simulink model "test_crypto_pc"  (R2019b)
settings: Solver=FixedStepAuto  StartTime=0.0  StopTime=20  FixedStep=0.0001  RelTol=1e-3
settings Model: Creator=Oboe  LastModifiedBy=Luca

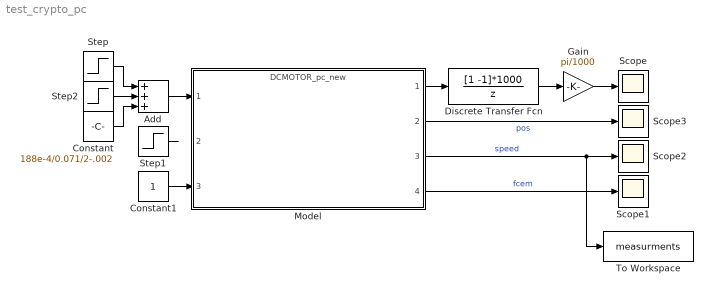
== system test_crypto_pc ==
  Add : Sum  Inputs=+++
  Constant : Constant  Value=188e-4/0.071/2-.002
  Constant1 : Constant
  Discrete Transfer Fcn : DiscreteTransferFcn  Numerator=[1 -1]*1000  Denominator=[1 0]  SampleTime=.001
  Gain : Gain  Gain=pi/1000
  Model : ModelReference  ModelNameDialog=DCMOTOR_pc_new.slxp  ModelReferenceVersion=1.21  CopyOfModelProtected=on
  Scope{,1..3} (4 alike) : Scope
  Step : Step  After=.5  SampleTime=0
  Step1 : Step  Time=10  After=-.5  SampleTime=0
  Step2 : Step  Time=10  After=-0.5  SampleTime=0
  To Workspace : ToWorkspace  VariableName=measurments  SaveFormat=Structure With Time  SampleTime=-1
      settings: Decimation=100
  wires:
  Model/1 -> Discrete Transfer Fcn/1
  Discrete Transfer Fcn/1 -> Gain/1
  Gain/1 -> Scope/1
  Model/4 -> Scope1/1  "fcem"
  Step/1 -> Add/1
  Constant/1 -> Add/3
  Step1/1 -> ?
  Model/2 -> Scope3/1  "pos"
  Model/3 -> To Workspace/1, Scope2/1  "speed"
  Add/1 -> Model/1
  Step2/1 -> Add/2
  Constant1/1 -> Model/3
